simulink model "simulink_model_advanced_closed_loop"  (R2018b)
settings: Solver=ode45  StartTime=0.0  StopTime=1  RelTol=1e-3
values from neighbouring files (symbols this model uses):
  N = 40    [extensive_example_ocp.m]    (also in minimal_example_closed_loop.m = 20; minimal_example_ocp.m = 20)
  nu = model.nu    [extensive_example_ocp.m]    (also in minimal_example_closed_loop.m; minimal_example_ocp.m; minimal_example_sim.m)
  nx = model.nx    [extensive_example_ocp.m]    (also in minimal_example_closed_loop.m; minimal_example_ocp.m; minimal_example_sim.m)
  ny = nu+nx    [extensive_example_ocp.m]    (also in minimal_example_ocp.m = size(model.cost_expr_y, 1))
  ny_e = nx    [extensive_example_ocp.m]    (also in minimal_example_ocp.m = size(model.cost_expr_y_e, 1))
  U_max = 80    [minimal_example_closed_loop.m]    (also in minimal_example_ocp.m)
  x0 = [0; pi; 0; 0]    [extensive_example_ocp.m]    (also in minimal_example_closed_loop.m = x_sim(:,i); minimal_example_ocp.m; minimal_example_sim.m = [0; 1e-1; 0; 0])
settings Model: Creator=oj  LastModifiedBy=oj
settings DataIOCC: SaveFormat=StructureWithTime  ReturnWorkspaceOutputs=on
settings OptimizationCC: LifeSpan=inf
settings DebuggingCC: FcnCallInpInsideContextMsg=warning  SFExecutionAtInitializationDiag=none
settings HardwareCC: ProdBitPerSizeT=32  ProdBitPerPtrDiffT=32  ProdWordSize=32  ProdHWDeviceType=Specified
settings CodeAppCC: StateflowObjectComments=on

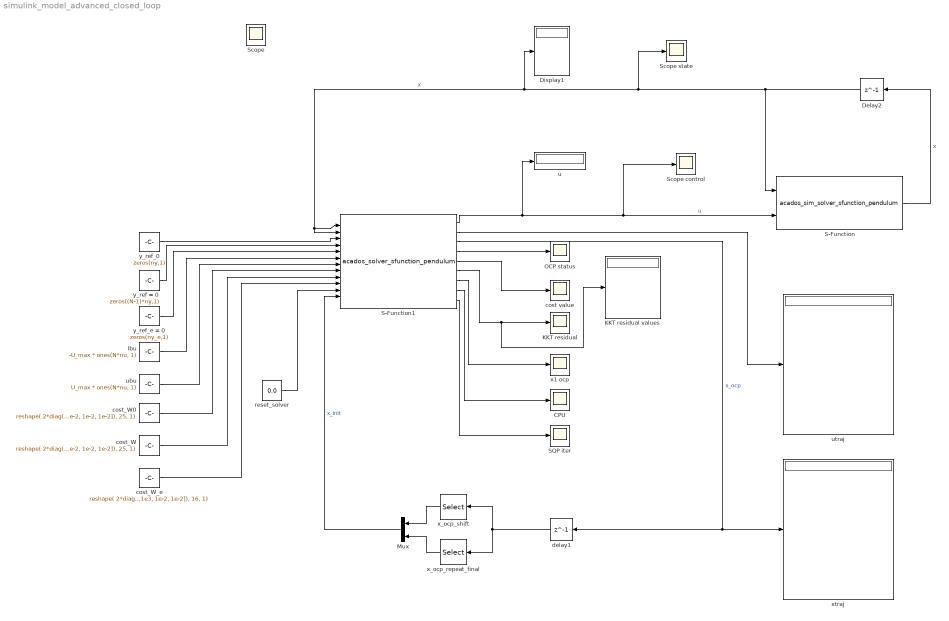
== system simulink_model_advanced_closed_loop ==
  CPU : Scope
      settings: Description=status
  Delay2 : Delay  DelayLength=1  InitialCondition=x0
  Display1 : Display
  KKT residual : Scope
      settings: Description=status
  KKT residual values : Display
  Mux : Mux  Inputs=2
  OCP status : Scope
      settings: Description=status
  S-Function : S-Function  FunctionName=acados_sim_solver_sfunction_pendulum  SFunctionDeploymentMode=off  EnableBusSupport=off
  S-Function1 : S-Function  FunctionName=acados_solver_sfunction_pendulum  SFunctionDeploymentMode=off  EnableBusSupport=off
  SQP iter : Scope
      settings: Description=status
  Scope control : Scope
  Scope state : Scope
  cost value : Scope
      settings: Description=status
  cost_W : Constant  Value=reshape( 2*diag([1e3, 1e3, 1e-2, 1e-2, 1e-2]), 25, 1)
  cost_W0 : Constant  Value=reshape( 2*diag([1e3, 1e3, 1e-2, 1e-2, 1e-2]), 25, 1)
  cost_W_e : Constant  Value=reshape( 2*diag([1e3, 1e3, 1e-2, 1e-2]), 16, 1)
  delay1 : Delay  DelayLength=1  InitialCondition=zeros(nx*(N+1),1)
  lbu : Constant  Value=-U_max * ones(N*nu, 1)
  reset_solver : Constant  Value=0.0
  u : Display
  ubu : Constant  Value=U_max * ones(N*nu, 1)
  utraj : Display
  x1 ocp : Scope
      settings: Description=status
  x_ocp_repeat_final : Selector  IndexMode=Zero-based  InputPortWidth=(N+1)*nx  IndexOptions=Starting index (dialog)  Indices=N*nx  OutputSizes=nx
  x_ocp_shift : Selector  IndexMode=Zero-based  InputPortWidth=(N+1)*nx  IndexOptions=Starting index (dialog)  Indices=nx  OutputSizes=N*nx
  xtraj : Display
  y_ref = 0 : Constant  Value=zeros((N-1)*ny,1)
  y_ref_0 : Constant  Value=zeros(ny,1)
  y_ref_e = 0 : Constant  Value=zeros(ny_e,1)
  Scope : Scope
  wires:
  S-Function/1 -> Delay2/1  "x"
  S-Function1/4 -> OCP status/1
  y_ref = 0/1 -> S-Function1/4
  y_ref_e = 0/1 -> S-Function1/5
  lbu/1 -> S-Function1/6
  ubu/1 -> S-Function1/7
  S-Function1/1 -> Scope control/1, S-Function/2, u/1  "u"
  Delay2/1 -> S-Function/1, Scope state/1, S-Function1/2, S-Function1/1, Display1/1  "x"
  cost_W0/1 -> S-Function1/8
  cost_W/1 -> S-Function1/9
  cost_W_e/1 -> S-Function1/10
  y_ref_0/1 -> S-Function1/3
  S-Function1/2 -> utraj/1
  x_ocp_shift/1 -> Mux/1
  delay1/1 -> x_ocp_shift/1, x_ocp_repeat_final/1
  Mux/1 -> S-Function1/12  "x_init"
  x_ocp_repeat_final/1 -> Mux/2
  S-Function1/3 -> xtraj/1, delay1/1  "x_ocp"
  reset_solver/1 -> S-Function1/11
  S-Function1/5 -> cost value/1
  S-Function1/6 -> KKT residual values/1, KKT residual/1
  S-Function1/7 -> x1 ocp/1
  S-Function1/8 -> CPU/1
  S-Function1/9 -> SQP iter/1
